simulink library "lib_affectiveChar_input"  (R2014a)
settings: Solver=ode45  StartTime=0.0  StopTime=10.0  RelTol=1e-3
undefined symbols (not defined in the file or in its folder): serial
libraries: simulink x3, instrumentlib x2
settings Model: Creator=Maryam  LastModifiedBy=Maryam

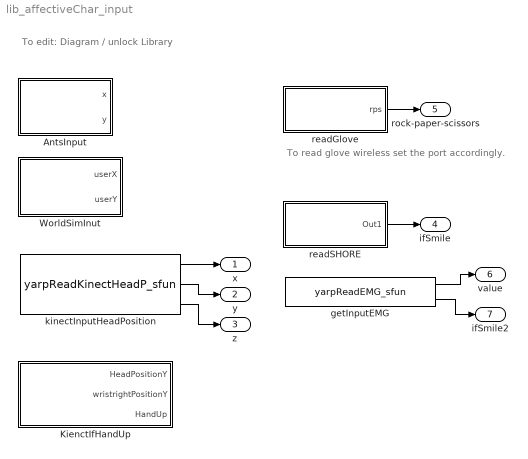
== system lib_affectiveChar_input ==
  note: To read glove wireless set the port accordingly.
  note: To edit: Diagram / unlock Library
  AntsInput : Subsystem
  KienctIfHandUp : Subsystem
  WorldSimInut : Subsystem
  getInputEMG : M-S-Function  FunctionName=yarpReadEMG_sfun  Parameters='/python/sending','/simulink/in1'
  kinectInputHeadPosition : M-S-Function  FunctionName=yarpReadKinectHeadP_sfun  Parameters='/mary/output','/simulink/in'
  readGlove : Subsystem
  readSHORE : Subsystem
  x : Outport
  y : Outport  Port=2
  z : Outport  Port=3
  ifSmile : Outport  Port=4
  rock-paper-scissors : Outport  Port=5
  value : Outport  Port=6
  ifSmile2 : Outport  Port=7
  wires:
  kinectInputHeadPosition/1 -> x/1
  kinectInputHeadPosition/2 -> y/1
  kinectInputHeadPosition/3 -> z/1
  readSHORE/1(Out1) -> ifSmile/1
  readGlove/1(rps) -> rock-paper-scissors/1
  getInputEMG/1 -> value/1
  getInputEMG/2 -> ifSmile2/1

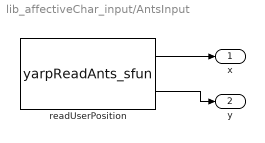
== system lib_affectiveChar_input/AntsInput ==
  readUserPosition : M-S-Function  FunctionName=yarpReadAnts_sfun  Parameters='/ants/out','/simulink/in'
  x : Outport
  y : Outport  Port=2
  wires:
  readUserPosition/1 -> x/1
  readUserPosition/2 -> y/1

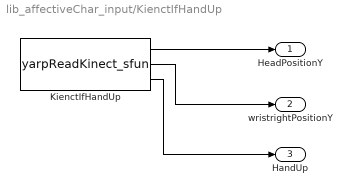
== system lib_affectiveChar_input/KienctIfHandUp ==
  KienctIfHandUp : M-S-Function  FunctionName=yarpReadKinect_sfun  Parameters='/mary/output','/simulink/in'
  HeadPositionY : Outport
  wristrightPositionY : Outport  Port=2
  HandUp : Outport  Port=3
  wires:
  KienctIfHandUp/1 -> HeadPositionY/1
  KienctIfHandUp/2 -> wristrightPositionY/1
  KienctIfHandUp/3 -> HandUp/1

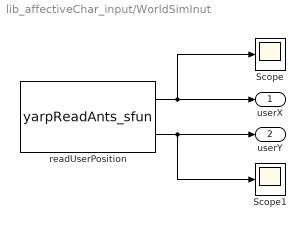
== system lib_affectiveChar_input/WorldSimInut ==
  Scope : Scope
  Scope1 : Scope
      settings: SaveName=ScopeData2
  readUserPosition : M-S-Function  FunctionName=yarpReadAnts_sfun  Parameters='/WS/actors/out','/simulink/in'
  userX : Outport
  userY : Outport  Port=2
  wires:
  readUserPosition/1 -> userX/1, Scope/1
  readUserPosition/2 -> Scope1/1, userY/1

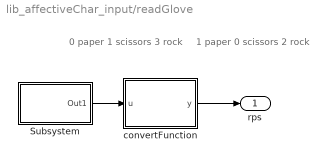
== system lib_affectiveChar_input/readGlove ==
  note: 0 paper
      | 1 scissors
      | 3 rock
  note: 1 paper
      | 0 scissors
      | 2 rock
  Subsystem : Subsystem
  convertFunction : MATLAB Function  TreatAsAtomicUnit=on
  rps : Outport
  wires:
  convertFunction/1(y) -> rps/1
  Subsystem/1(Out1) -> convertFunction/1(u)

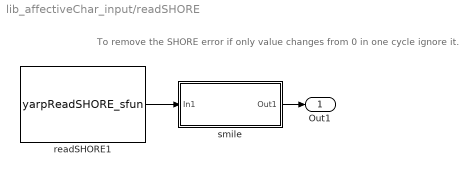
== system lib_affectiveChar_input/readSHORE ==
  note: To remove the SHORE error if only value changes from 0 in one cycle ignore it.
  readSHORE1 : M-S-Function  FunctionName=yarpReadSHORE_sfun  Parameters='/testSender','/simulink/in'
  smile : Subsystem
  Out1 : Outport
  wires:
  readSHORE1/1 -> smile/1(In1)
  smile/1(Out1) -> Out1/1

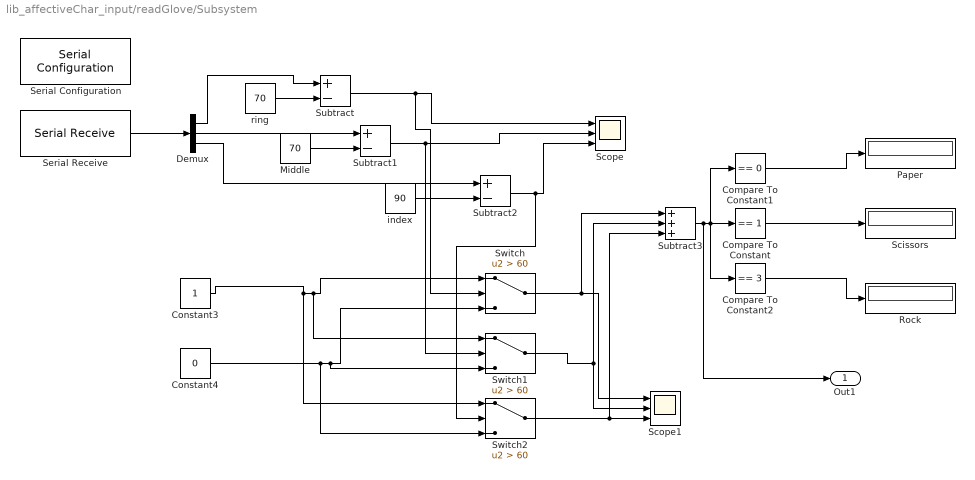
== system lib_affectiveChar_input/readGlove/Subsystem ==
  Compare To Constant : simulink/Logic and Bit Operations/Compare To Constant  relop===  const=1  OutDataTypeStr=boolean
  Compare To Constant1 : simulink/Logic and Bit Operations/Compare To Constant  relop===  const=0  OutDataTypeStr=boolean
  Compare To Constant2 : simulink/Logic and Bit Operations/Compare To Constant  relop===  const=3  OutDataTypeStr=boolean
  Constant3 : Constant
  Constant4 : Constant  Value=0
  Demux : Demux  Outputs=3
  Middle : Constant  Value=70
  Paper : Display
  Rock : Display
  Scissors : Display
  Scope : Scope  NumInputPorts=3
      settings: YMin=-25~20~-25  YMax=200~200~200
  Scope1 : Scope  NumInputPorts=3
      settings: YMin=-0.5~-0.5~-1  YMax=1.5~1.5~1.5
  Serial Configuration : instrumentlib/Serial Configuration  Priority=-200000  ComPortMenu=COM4  ComPort=COM4  ObjConstructor=serial('COM4');  BaudRate=9600  DataBits=8  Parity=none  StopBits=1  FlowControl=none  Timeout=10  ByteOrder=LittleEndian
  Serial Receive : instrumentlib/Serial Receive  ComPortMenu=COM4  ComPort=COM4  ObjConstructor=serial('COM4');  Terminator=<none>  DataSize="[3  1]"  DataType=uint8  EnableBlockingMode=on  ActionDataUnavailable=Output last received value  CustomValue=0  SampleTime=0.01
  Subtract : Sum  Inputs=+-
  Subtract1 : Sum  Inputs=+-
  Subtract2 : Sum  Inputs=+-
  Subtract3 : Sum  Inputs=+++
  Switch : Switch  Criteria=u2 > Threshold  Threshold=60
  Switch1 : Switch  Criteria=u2 > Threshold  Threshold=60
  Switch2 : Switch  Criteria=u2 > Threshold  Threshold=60
  index : Constant  Value=90
  ring : Constant  Value=70
  Out1 : Outport
  wires:
  Serial Receive/1 -> Demux/1
  Compare To Constant2/1 -> Rock/1
  Compare To Constant/1 -> Scissors/1
  Compare To Constant1/1 -> Paper/1
  Subtract3/1 -> Compare To Constant1/1, Compare To Constant2/1, Compare To Constant/1, Out1/1
  Switch2/1 -> Scope1/3, Subtract3/3
  Switch1/1 -> Scope1/2, Subtract3/2
  Constant4/1 -> Switch/3, Switch1/3, Switch2/3
  Constant3/1 -> Switch/1, Switch1/1, Switch2/1
  Switch/1 -> Scope1/1, Subtract3/1
  index/1 -> Subtract2/2
  Middle/1 -> Subtract1/2
  ring/1 -> Subtract/2
  Subtract1/1 -> Scope/2, Switch1/2
  Subtract2/1 -> Scope/3, Switch2/2
  Subtract/1 -> Scope/1, Switch/2
  Demux/3 -> Subtract2/1
  Demux/2 -> Subtract1/1
  Demux/1 -> Subtract/1

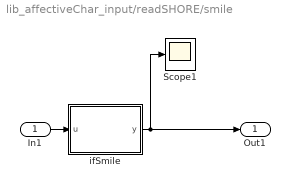
== system lib_affectiveChar_input/readSHORE/smile ==
  In1 : Inport
  Scope1 : Scope
      settings: SaveName=ScopeData3
  ifSmile : MATLAB Function  TreatAsAtomicUnit=on
  Out1 : Outport
  wires:
  In1/1 -> ifSmile/1(u)
  ifSmile/1(y) -> Scope1/1, Out1/1

== matlab function lib_affectiveChar_input/readGlove/convertFunction ==
  data: u input; y output
function y = fcn(u)
%#codegen
%    paper=0; 'rock'=3;'scissors'=1;
%to 'paper'=1;'rock'=2;'scissors'=0;

if(u==0)
    u=1;
elseif(u==1)
    u=0;
elseif(u==3)
    u=2;
else 
    u=3;
end
y = u;

== matlab function lib_affectiveChar_input/readSHORE/smile/ifSmile ==
  data: u input; y output
function y = fcn(u)
%#codegen
if u>10
    smile=1;
else
    smile=0;
end
y = smile;
